simulink model "BoostConverter_Example"  (R2020b)
settings: Solver=FixedStepAuto  StartTime=0.0  StopTime=100  FixedStep=0.0015  RelTol=1e-3
libraries: PB_Library_Master x1, Lib_Solve_SSNRSolverJC_EMTAT x1
settings Model: Creator=pmatt  LastModifiedBy=nbutler2
settings SFSimCC: CustomCodeUndefinedFunction=UseInterfaceOnly

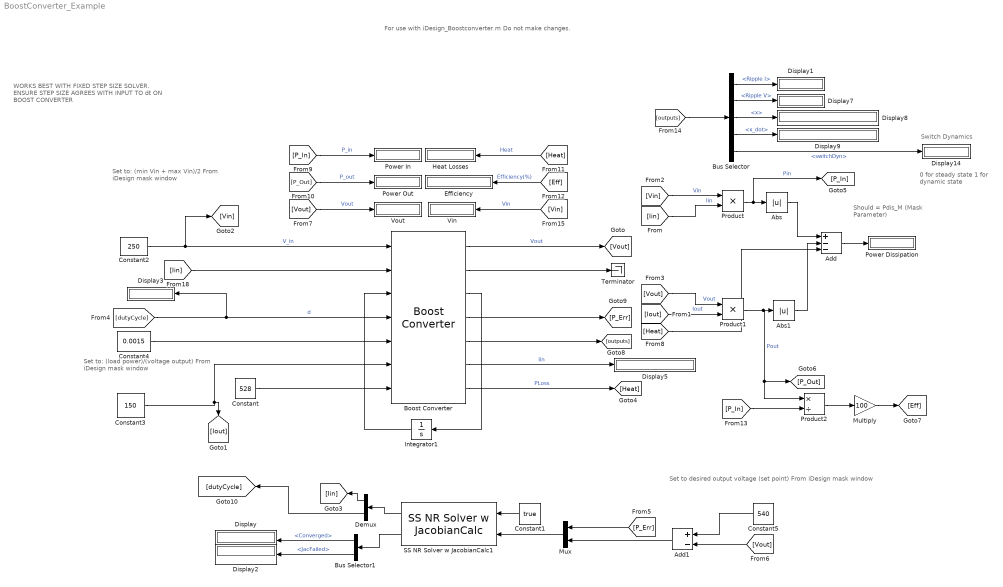
== system BoostConverter_Example ==
  note: WORKS BEST WITH FIXED
      | STEP SIZE SOLVER. ENSURE
      | STEP SIZE AGREES WITH INPUT
      | TO dt ON BOOST CONVERTER
  note: Set to:
      | (load power)/(voltage output)
      | From iDesign mask window
  note: Set to desired output voltage (set point)
      | From iDesign mask window
  note: Switch Dynamics
  note: Should = Pdis_M
      | (Mask Parameter)
  note: For use with iDesign_Boostconverter.m
      | Do not make changes.
  note: 0 for steady state
      | 1 for dynamic state
  note: Set to:
      | (min Vin + max Vin)/2
      | From iDesign mask window
  Abs : Abs
  Abs1 : Abs
  Add : Sum  Inputs=+--
  Add1 : Sum  Inputs=+-
  Boost Converter : PB_Library_Master/Boost Converter  Pdis_M=1  C_M=1.65e-07  L_M=0.00022824  Ron_M=0.036  RC_M=0.037475  RL_M=0.072284  QgTotal_M=8.4e-08  Vdiode_M=1.2  TRise_M=1.72e-07  TFall_M=7.8e-08  Fsw_M=250000  Vgate_M=4  n_MOSFET=1  MassEst_M=18.7575  TempIn=Celsius  vOut=540  pow=5000  minV=240  maxV=260  rippleMode=Use defaults (5% of voltage output and 10% of inductor current)  vRip=.05  iRip=.1  freqMode=Use default frequency (250 kHz)  freq=250e3
  Bus Selector : BusSelector  OutputSignals=Ripple I,Ripple V,x,x_dot,switchDyn
  Bus Selector1 : BusSelector  OutputSignals=Converged,JacFailed
  Constant : Constant  Value=528
  Constant1 : Constant  Value=true
  Constant2 : Constant  Value=250  VectorParams1D=off  SampleTime=-1
  Constant3 : Constant  Value=150
  Constant4 : Constant  Value=0.0015  VectorParams1D=off
  Constant5 : Constant  Value=540
  Demux : Demux  Outputs=2
  Display{,1..3,5,7..9,14} (9 alike) : Display
      Display8 settings: Decimation=3
  Efficiency : Display
  Heat Losses : Display
  Integrator1 : Integrator  InitialCondition=[0;0]
  Multiply : Gain  Gain=100
  Mux : Mux  Inputs=2
  Power Dissipation : Display
  Power In : Display
  Power Out : Display
  Product : Product
  Product1 : Product
  Product2 : Product  Inputs=*/
  SS NR Solver w JacobianCalc1 : Lib_Solve_SSNRSolverJC_EMTAT/SS NR Solver w JacobianCalc  SJac_Per_M=.01 * [1 -1; 1 -1]  SNR_IC_M=[1;.5]  SNR_DX_M=10  SNR_Mx_M=[100000;.99999]  SNR_Mn_M=[0.00001;.0001]  SJacobianAttempts_M=200  Cond_Limits_M=0.0001
  Terminator : Terminator
  Vin : Display
  Vout : Display
  wires:
  [Iin] -> Boost Converter/2
  [Eff] -> Efficiency/1  "Efficiency(%)"
  Integrator1/1 -> Boost Converter/3
  Boost Converter/5 -> [outputs]
  [Vout] -> Product1/1  "Vout"
  Constant2/1 -> Boost Converter/1, [Vin]  "V_in"
  Bus Selector/2 -> Display7/1  "<Ripple V>"
  Bus Selector/5 -> Display14/1  "<switchDyn>"
  Bus Selector/4 -> Display9/1  "<x_dot>"
  Boost Converter/7 -> [Heat]  "PLoss"
  [Iin] -> Product/2  "Iin"
  Boost Converter/6 -> Display5/1  "Iin"
  [Iout] -> Product1/2  "Iout"
  [P_Out] -> Power Out/1  "P_out"
  Abs1/1 -> Add/2
  Abs/1 -> Add/1
  [outputs] -> Bus Selector/1
  Bus Selector/1 -> Display1/1  "<Ripple I>"
  Boost Converter/3 -> Integrator1/1
  [Vin] -> Product/1  "Vin"
  [Heat] -> Heat Losses/1  "Heat"
  Bus Selector/3 -> Display8/1  "<x>"
  [P_In] -> Product2/2
  Add/1 -> Power Dissipation/1
  Product/1 -> [P_In], Abs/1  "Pin"
  Boost Converter/1 -> [Vout]  "Vout"
  Multiply/1 -> [Eff]
  Product2/1 -> Multiply/1
  [P_In] -> Power In/1  "P_in"
  Product1/1 -> [P_Out], Product2/1, Abs1/1  "Pout"
  Constant/1 -> Boost Converter/7
  Boost Converter/2 -> Terminator/1
  Constant3/1 -> Boost Converter/6, [Iout]
  [Heat] -> Add/3
  Constant4/1 -> Boost Converter/5
  [dutyCycle] -> Boost Converter/4, Display3/1  "d"
  Constant1/1 -> SS NR Solver w JacobianCalc1/1
  SS NR Solver w JacobianCalc1/2 -> Bus Selector1/1
  Bus Selector1/1 -> Display/1  "<Converged>"
  Bus Selector1/2 -> Display2/1  "<JacFailed>"
  [Vout] -> Add1/2
  Constant5/1 -> Add1/1
  Add1/1 -> Mux/2
  Mux/1 -> SS NR Solver w JacobianCalc1/2
  [P_Err] -> Mux/1
  SS NR Solver w JacobianCalc1/1 -> Demux/1
  Demux/1 -> [Iin]
  Demux/2 -> [dutyCycle]
  [Vout] -> Vout/1  "Vout"
  [Vin] -> Vin/1  "Vin"
  Boost Converter/4 -> [P_Err]
